simulink model "force_alone"  (R2020a)
settings: Solver=ode15s  StartTime=0.0  StopTime=8  FixedStep=1e-3  RelTol=1e-2  AbsTol=1e-2
values from neighbouring files (symbols this model uses):
  Fd = [0 0 9 0 0 0]    [JoinScript.m]    (also in alldata.mat)
  InvMd = inv(Md)    [JoinScript.m]    (also in alldata.mat = [0.01 0 0 0 0 0 0 0.01 0 0 0 0 ... (36 elements, 6x6)])
  K = [C11 C12 C13 0 0 0; C12 C11 C13 0 0 0; C13 C13 C33 0 0 0; 0 0 0 C44 0 0; 0 0 0 0 C44 0; 0 0 0 0 0 C66]    [JoinScript.m]    (also in alldata.mat = [20.1 11.1 12 0 0 0 11.1 20.1 12 0 0 0 ... (36 elements, 6x6; aux_y2.m = Abb.fkine(q))
  Kd = 150*diag([1 1 1 1 1 1])    [JoinScript.m]    (also in alldata.mat = [150 0 0 0 0 0 0 150 0 0 0 0 ... (36 elements, 6x6)]; aux_y.m = 3e2*diag([1 1 1 1 1 1]); aux_y2.m = 3e2*diag([1 1 1 1 1 1]))
  Kp = 200*diag([1 1 1 1 1 1])    [JoinScript.m]    (also in alldata.mat = [200 0 0 0 0 0 0 200 0 0 0 0 ... (36 elements, 6x6)]; aux_y.m = 1e3*diag([1 1 1 1 1 1]); aux_y2.m = 1e3*diag([1 1 1 1 1 1]))
  qf = [pi/2 pi/3 pi/12 pi/2 0 pi/2]    [JoinScript.m]    (also in alldata.mat = [1.57079632679 1.0471975512 0.261799387799 1.57079632679 0 1; model_script.m = [pi/6 0 pi/3 pi/4 0 0])
  x0 = dir_kin(qf)    [JoinScript.m]    (also in alldata.mat = [-5.32301496588e-18 0.480120382501 0.16494818601 1.570796326)
settings Model: SimulationMode=accelerator  Creator=doble  LastModifiedBy=doble
settings SolverCC: InitialStep=1e-3  MaxOrder=3  ZeroCrossControl=EnableAll

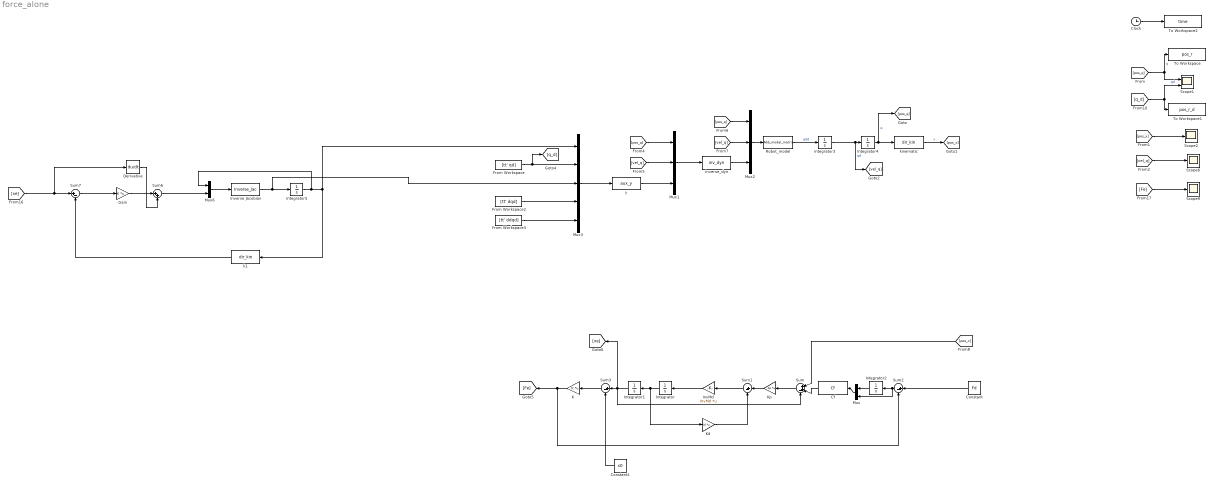
== system force_alone ==
  Cf : MATLABFcn  MATLABFcn=Cf  OutputDimensions=6*1
  Clock : Clock
      settings: Decimation=18
  Constant : Constant  Value=Fd
  Constant1 : Constant  Value=x0
  Derivative : Derivative
  From Workspace : FromWorkspace  VariableName=[tt' qd]
  From Workspace2 : FromWorkspace  VariableName=[tt' dqd]
  From Workspace3 : FromWorkspace  VariableName=[tt' ddqd]
  Gain : Gain  Gain=K  Multiplication=Matrix(K*u)
  Integrator : Integrator
  Integrator1 : Integrator  InitialCondition=x0
  Integrator2 : Integrator
  Integrator3 : Integrator
  Integrator4 : Integrator  InitialCondition=qf
  Integrator5 : Integrator  InitialCondition=qf
  InvMd : Gain  Gain=InvMd  Multiplication=Matrix(K*u)
  Inverse Jacobian : MATLABFcn  MATLABFcn=Inverse_Jac  OutputDimensions=6*1
  K : Gain  Gain=K  Multiplication=Matrix(K*u)
  Kd : Gain  Gain=Kd  Multiplication=Matrix(K*u)
  Kp : Gain  Gain=Kp  Multiplication=Matrix(K*u)
  Mux : Mux  Inputs=2
  Mux1 : Mux  Inputs=[6 6 6]
  Mux2 : Mux  Inputs=[6 6 6]
  Mux3 : Mux  Inputs=[6 6 6 6 6]
  Mux6 : Mux  Inputs=[6 6]
  Robot_model : MATLABFcn  MATLABFcn=Abb_model_matrix  OutputDimensions=6
  Scope1 : Scope  NumInputPorts=2
  Scope2 : Scope
  Scope6 : Scope
  Scope9 : Scope
  Sum : Sum  Inputs=|++-
  Sum{1..3,7} (4 alike) : Sum  Inputs=|+-
  Sum6 : Sum  Inputs=|++
  To Workspace : ToWorkspace  VariableName=pos_r  SampleTime=-1
  To Workspace1 : ToWorkspace  VariableName=pos_r_d  SampleTime=-1
  To Workspace2 : ToWorkspace  VariableName=time  SampleTime=-1
  inverse_dyn : MATLABFcn  MATLABFcn=inv_dyn  OutputDimensions=6
  k1 : MATLABFcn  MATLABFcn=dir_kin
  kinematic : MATLABFcn  MATLABFcn=dir_kin
  y : MATLABFcn  MATLABFcn=aux_y
  wires:
  K/1 -> [Fe], Sum2/2
  From Workspace/1 -> Mux3/2, [q_d]
  [xe] -> Derivative/1, Sum7/1
  [pos_q] -> To Workspace/1, Scope1/1  "q"
  [pos_x] -> Sum/1
  Mux1/1 -> inverse_dyn/1
  Integrator3/1 -> [vel_q], Integrator4/1  "qd"
  Mux6/1 -> Inverse Jacobian/1
  Sum6/1 -> Mux6/2
  Sum2/1 -> Integrator2/1, Mux/2
  Gain/1 -> Sum6/1
  Integrator1/1 -> Sum/3, [xe], Sum3/1
  Sum7/1 -> Gain/1
  [pos_x] -> Scope2/1
  [q_d] -> To Workspace1/1, Scope1/2  "qd"
  Derivative/1 -> Sum6/2
  [vel_q] -> Mux2/2
  Mux3/1 -> y/1
  inverse_dyn/1 -> Mux2/3
  Robot_model/1 -> Integrator3/1  "qdd"
  kinematic/1 -> [pos_x]  "x"
  Inverse Jacobian/1 -> Mux3/3, Integrator5/1
  Sum3/1 -> K/1
  From Workspace2/1 -> Mux3/4
  Sum/1 -> Kp/1
  Constant1/1 -> Sum3/2
  [vel_q] -> Scope6/1
  [pos_q] -> Mux1/1
  Constant/1 -> Sum2/1
  [Fe] -> Scope9/1
  Integrator/1 -> Kd/1, Integrator1/1
  From Workspace3/1 -> Mux3/5
  Sum1/1 -> InvMd/1
  Integrator2/1 -> Mux/1
  Integrator5/1 -> Mux6/1, Mux3/1, k1/1
  k1/1 -> Sum7/2
  y/1 -> Mux1/3
  Kp/1 -> Sum1/1
  [vel_q] -> Mux1/2
  Mux2/1 -> Robot_model/1
  Cf/1 -> Sum/2
  Kd/1 -> Sum1/2
  [pos_q] -> Mux2/1
  Integrator4/1 -> [pos_q], kinematic/1  "q"
  Mux/1 -> Cf/1
  Clock/1 -> To Workspace2/1
  InvMd/1 -> Integrator/1
